simulink model "Lombardini_dual_fuel"  (R2024b)
settings: Solver=FixedStepAuto  StartTime=0.0  StopTime=2000  RelTol=1e-3  EnableMultiTasking=on
PreLoadFcn:
  | try, eval([bdroot '_setup']); catch, eval('model_setup', ''); end
InitFcn:
  | try, eval([bdroot '_setup']); catch, eval('model_setup', ''); end
model workspace (MAT data in the model file):
  PID_rpm = [1000 2000 3000 4000]
undefined symbols (not defined in the file): ECU555, motohawk_build_version, motohawk_get_target_image, motohawk_target_type, motohawk_trunc_name, motohawk_vardec_path
libraries: MotoHawk_lib x118, motohawk_annotations_lib x23, dspstat3 x13, motohawk_examples_lib x1, MotoHawk_Protocols_lib x1
(part 3 of 5)

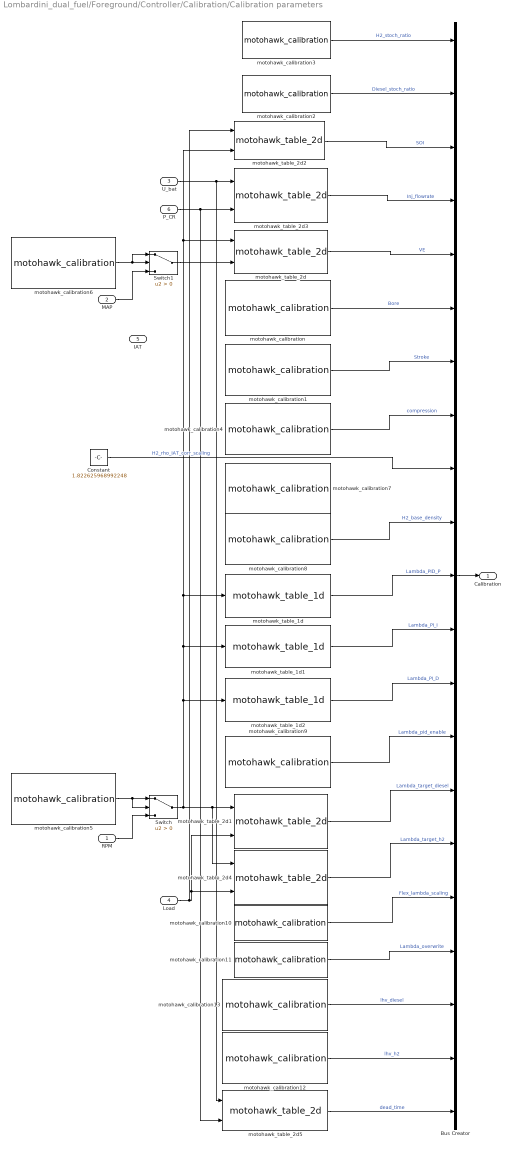
== system Lombardini_dual_fuel/Foreground/Controller/Calibration/Calibration parameters ==
  RPM : Inport
  MAP : Inport  Port=2
  U_bat : Inport  Port=3
  Load : Inport  Port=4
  IAT : Inport  Port=5
  P_CR : Inport  Port=6
  Bus Creator : BusCreator  Inputs=21
  Constant : Constant  Value=1.822625968992248
  Switch : Switch  Criteria=u2 > Threshold  SaturateOnIntegerOverflow=off  InputSameDT=off
  Switch1 : Switch  Criteria=u2 > Threshold  SaturateOnIntegerOverflow=off  InputSameDT=off
  motohawk_calibration : MotoHawk_lib/Calibration & Probing Blocks/motohawk_calibration  name_source=Use Parameter  nam='Bore'  val=69  storage=Calibration  ovr_cals=on  data_type=Inherit from 'Default Value'  mem_region_use=off  mem_region_name='SERIAL_EE'  read_level=1  write_level=1  view_as=Number  enum_struct={'Disabled', 'Enabled'}  vector_style=Wide Row  row_header_enum={}  col_header_enum={}  mototune_group=motohawk_vardec_path(gcb)  help=''  units=''  min_val=-inf  max_val=inf  precision=''  gain=1  offset=0  exp=1  show_more=on  use_help_units=on  use_header_enum=off  use_min_max=off  use_precision=off  use_mototune_group=on  data_stores=motohawk_sfun_calibration_data_stores
      settings: SourceProductName=MotoHawk
  motohawk_calibration1 : MotoHawk_lib/Calibration & Probing Blocks/motohawk_calibration  name_source=Use Parameter  nam='Stroke'  val=64  storage=Calibration  ovr_cals=on  data_type=Inherit from 'Default Value'  mem_region_use=off  mem_region_name='SERIAL_EE'  read_level=1  write_level=1  view_as=Number  enum_struct={'Disabled', 'Enabled'}  vector_style=Wide Row  row_header_enum={}  col_header_enum={}  mototune_group=motohawk_vardec_path(gcb)  help=''  units=''  min_val=-inf  max_val=inf  precision=''  gain=1  offset=0  exp=1  show_more=on  use_help_units=on  use_header_enum=off  use_min_max=off  use_precision=off  use_mototune_group=on  data_stores=motohawk_sfun_calibration_data_stores
      settings: SourceProductName=MotoHawk
  motohawk_calibration10 : MotoHawk_lib/Calibration & Probing Blocks/motohawk_calibration  name_source=Use Parameter  nam='Flex_lambda_scaling'  val=1  storage=Calibration  ovr_cals=on  data_type=Inherit from 'Default Value'  mem_region_use=off  mem_region_name='SERIAL_EE'  read_level=1  write_level=1  view_as=Number  enum_struct={'Disabled', 'Enabled'}  vector_style=Wide Row  row_header_enum={}  col_header_enum={}  mototune_group=motohawk_vardec_path(gcb)  help=''  units=''  min_val=-inf  max_val=inf  precision=''  gain=1  offset=0  exp=1  show_more=off  use_help_units=off  use_header_enum=off  use_min_max=off  use_precision=off  use_mototune_group=off  data_stores=motohawk_sfun_calibration_data_stores
      settings: SourceProductName=MotoHawk
  motohawk_calibration11 : MotoHawk_lib/Calibration & Probing Blocks/motohawk_calibration  name_source=Use Parameter  nam='Lambda_Overwrite'  val=0  storage=Calibration  ovr_cals=on  data_type=Inherit from 'Default Value'  mem_region_use=off  mem_region_name='SERIAL_EE'  read_level=1  write_level=1  view_as=Number  enum_struct={'Disabled', 'Enabled'}  vector_style=Wide Row  row_header_enum={}  col_header_enum={}  mototune_group=motohawk_vardec_path(gcb)  help=''  units=''  min_val=-inf  max_val=inf  precision=''  gain=1  offset=0  exp=1  show_more=off  use_help_units=off  use_header_enum=off  use_min_max=off  use_precision=off  use_mototune_group=off  data_stores=motohawk_sfun_calibration_data_stores
      settings: SourceProductName=MotoHawk
  motohawk_calibration12 : MotoHawk_lib/Calibration & Probing Blocks/motohawk_calibration  name_source=Use Parameter  nam='LHV_H2'  val=120000  storage=Calibration  ovr_cals=on  data_type=Inherit from 'Default Value'  mem_region_use=off  mem_region_name='SERIAL_EE'  read_level=1  write_level=1  view_as=Number  enum_struct={'Disabled', 'Enabled'}  vector_style=Wide Row  row_header_enum={}  col_header_enum={}  mototune_group=motohawk_vardec_path(gcb)  help=''  units=''  min_val=-inf  max_val=inf  precision=''  gain=1  offset=0  exp=1  show_more=on  use_help_units=on  use_header_enum=off  use_min_max=off  use_precision=off  use_mototune_group=on  data_stores=motohawk_sfun_calibration_data_stores
      settings: SourceProductName=MotoHawk
  motohawk_calibration13 : MotoHawk_lib/Calibration & Probing Blocks/motohawk_calibration  name_source=Use Parameter  nam='LHV_Diesel'  val=42800  storage=Calibration  ovr_cals=on  data_type=Inherit from 'Default Value'  mem_region_use=off  mem_region_name='SERIAL_EE'  read_level=1  write_level=1  view_as=Number  enum_struct={'Disabled', 'Enabled'}  vector_style=Wide Row  row_header_enum={}  col_header_enum={}  mototune_group=motohawk_vardec_path(gcb)  help=''  units=''  min_val=-inf  max_val=inf  precision=''  gain=1  offset=0  exp=1  show_more=on  use_help_units=on  use_header_enum=off  use_min_max=off  use_precision=off  use_mototune_group=on  data_stores=motohawk_sfun_calibration_data_stores
      settings: SourceProductName=MotoHawk
  motohawk_calibration2 : MotoHawk_lib/Calibration & Probing Blocks/motohawk_calibration  name_source=Use Parameter  nam='Diesel_Stoch_ratio'  val=14.7  storage=Calibration  ovr_cals=on  data_type=Inherit from 'Default Value'  mem_region_use=off  mem_region_name='SERIAL_EE'  read_level=1  write_level=1  view_as=Number  enum_struct={'Disabled', 'Enabled'}  vector_style=Wide Row  row_header_enum={}  col_header_enum={}  mototune_group=motohawk_vardec_path(gcb)  help=''  units=''  min_val=-inf  max_val=inf  precision=''  gain=1  offset=0  exp=1  show_more=off  use_help_units=off  use_header_enum=off  use_min_max=off  use_precision=off  use_mototune_group=off  data_stores=motohawk_sfun_calibration_data_stores
      settings: SourceProductName=MotoHawk
  motohawk_calibration3 : MotoHawk_lib/Calibration & Probing Blocks/motohawk_calibration  name_source=Use Parameter  nam='H2_Stoch_ratio'  val=34.3  storage=Calibration  ovr_cals=on  data_type=Inherit from 'Default Value'  mem_region_use=off  mem_region_name='SERIAL_EE'  read_level=1  write_level=1  view_as=Number  enum_struct={'Disabled', 'Enabled'}  vector_style=Wide Row  row_header_enum={}  col_header_enum={}  mototune_group=motohawk_vardec_path(gcb)  help=''  units=''  min_val=-inf  max_val=inf  precision=''  gain=1  offset=0  exp=1  show_more=off  use_help_units=off  use_header_enum=off  use_min_max=off  use_precision=off  use_mototune_group=off  data_stores=motohawk_sfun_calibration_data_stores
      settings: SourceProductName=MotoHawk
  motohawk_calibration4 : MotoHawk_lib/Calibration & Probing Blocks/motohawk_calibration  name_source=Use Parameter  nam='Compression'  val=20  storage=Calibration  ovr_cals=on  data_type=Inherit from 'Default Value'  mem_region_use=off  mem_region_name='SERIAL_EE'  read_level=1  write_level=1  view_as=Number  enum_struct={'Disabled', 'Enabled'}  vector_style=Wide Row  row_header_enum={}  col_header_enum={}  mototune_group=motohawk_vardec_path(gcb)  help=''  units=''  min_val=-inf  max_val=inf  precision=''  gain=1  offset=0  exp=1  show_more=on  use_help_units=on  use_header_enum=off  use_min_max=off  use_precision=off  use_mototune_group=on  data_stores=motohawk_sfun_calibration_data_stores
      settings: SourceProductName=MotoHawk
  motohawk_calibration5 : MotoHawk_lib/Calibration & Probing Blocks/motohawk_calibration  name_source=Use Parameter  nam='RPM_Overwrite'  val=0  storage=Calibration  ovr_cals=on  data_type=Inherit from 'Default Value'  mem_region_use=off  mem_region_name='SERIAL_EE'  read_level=1  write_level=1  view_as=Number  enum_struct={'Disabled', 'Enabled'}  vector_style=Wide Row  row_header_enum={}  col_header_enum={}  mototune_group=motohawk_vardec_path(gcb)  help=''  units=''  min_val=-inf  max_val=inf  precision=''  gain=1  offset=0  exp=1  show_more=on  use_help_units=on  use_header_enum=off  use_min_max=off  use_precision=off  use_mototune_group=on  data_stores=motohawk_sfun_calibration_data_stores
      settings: SourceProductName=MotoHawk
  motohawk_calibration6 : MotoHawk_lib/Calibration & Probing Blocks/motohawk_calibration  name_source=Use Parameter  nam='MAP_Overwrite'  val=0  storage=Calibration  ovr_cals=on  data_type=Inherit from 'Default Value'  mem_region_use=off  mem_region_name='SERIAL_EE'  read_level=1  write_level=1  view_as=Number  enum_struct={'Disabled', 'Enabled'}  vector_style=Wide Row  row_header_enum={}  col_header_enum={}  mototune_group=motohawk_vardec_path(gcb)  help=''  units=''  min_val=-inf  max_val=inf  precision=''  gain=1  offset=0  exp=1  show_more=on  use_help_units=on  use_header_enum=off  use_min_max=off  use_precision=off  use_mototune_group=on  data_stores=motohawk_sfun_calibration_data_stores
      settings: SourceProductName=MotoHawk
  motohawk_calibration7 : MotoHawk_lib/Calibration & Probing Blocks/motohawk_calibration  name_source=Use Parameter  nam='H2_rho_IAT_corr_gain'  val=1.5  storage=Calibration  ovr_cals=on  data_type=Inherit from 'Default Value'  mem_region_use=off  mem_region_name='SERIAL_EE'  read_level=1  write_level=1  view_as=Number  enum_struct={'Disabled', 'Enabled'}  vector_style=Wide Row  row_header_enum={}  col_header_enum={}  mototune_group=motohawk_vardec_path(gcb)  help=''  units=''  min_val=-inf  max_val=inf  precision=''  gain=1  offset=0  exp=1  show_more=on  use_help_units=on  use_header_enum=off  use_min_max=off  use_precision=off  use_mototune_group=on  data_stores=motohawk_sfun_calibration_data_stores
      settings: SourceProductName=MotoHawk
  motohawk_calibration8 : MotoHawk_lib/Calibration & Probing Blocks/motohawk_calibration  name_source=Use Parameter  nam='H2_base_density'  val=0.00008988  storage=Calibration  ovr_cals=on  data_type=Inherit from 'Default Value'  mem_region_use=off  mem_region_name='SERIAL_EE'  read_level=1  write_level=1  view_as=Number  enum_struct={'Disabled', 'Enabled'}  vector_style=Wide Row  row_header_enum={}  col_header_enum={}  mototune_group=motohawk_vardec_path(gcb)  help=''  units=''  min_val=-inf  max_val=inf  precision=''  gain=1  offset=0  exp=1  show_more=on  use_help_units=on  use_header_enum=off  use_min_max=off  use_precision=off  use_mototune_group=on  data_stores=motohawk_sfun_calibration_data_stores
      settings: SourceProductName=MotoHawk
  motohawk_calibration9 : MotoHawk_lib/Calibration & Probing Blocks/motohawk_calibration  name_source=Use Parameter  nam='Lambda_pid_enable'  val=0  storage=Calibration  ovr_cals=on  data_type=Inherit from 'Default Value'  mem_region_use=off  mem_region_name='SERIAL_EE'  read_level=1  write_level=1  view_as=Number  enum_struct={'Disabled', 'Enabled'}  vector_style=Wide Row  row_header_enum={}  col_header_enum={}  mototune_group=motohawk_vardec_path(gcb)  help=''  units=''  min_val=-inf  max_val=inf  precision=''  gain=1  offset=0  exp=1  show_more=on  use_help_units=on  use_header_enum=off  use_min_max=off  use_precision=off  use_mototune_group=on  data_stores=motohawk_sfun_calibration_data_stores
      settings: SourceProductName=MotoHawk
  motohawk_table_1d : MotoHawk_lib/Lookup Tables/motohawk_table_1d  nam='Lambda_PID_P'  bp_nam=''  breakpoint_data=PID_rpm  bp_data_type=Inherit from 'Breakpoint Data'  table_data=[0.5 0.5 0.5 0.5]  table_data_type=Inherit from 'Table Data'  out_type=Inherit from 'Table Data'  input_name=''  output_name=''  bp_storage=Constant  bp_mem_region_use=off  bp_mem_region_name='SERIAL_EE'  storage=NonAdaptive  mem_region_use=off  mem_region_name='SERIAL_EE'  read_level=1  write_level=1  ovr_cals=on  mototune_group=motohawk_vardec_path(gcb)  help=''  bp_units=''  table_units=''  bp_min_val=-inf  bp_max_val=inf  min_val=-inf  max_val=inf  b_precision=''  b_gain=1  b_offset=0  b_exp=1  t_precision=''  t_gain=1  t_offset=0  t_exp=1  show_more=on  use_help=off  use_min_max=off  use_precision=off  use_breakpoint=off  use_table=off  use_links=off  use_mototune_group=off  data_stores=motohawk_table_1d_data_stores
      settings: SourceProductName=MotoHawk
  motohawk_table_1d1 : MotoHawk_lib/Lookup Tables/motohawk_table_1d  nam='Lambda_PID_I'  bp_nam=''  breakpoint_data=PID_rpm  bp_data_type=Inherit from 'Breakpoint Data'  table_data=[0.5 0.5 0.5 0.5 ]  table_data_type=Inherit from 'Table Data'  out_type=Inherit from 'Table Data'  input_name=''  output_name=''  bp_storage=Constant  bp_mem_region_use=off  bp_mem_region_name='SERIAL_EE'  storage=NonAdaptive  mem_region_use=off  mem_region_name='SERIAL_EE'  read_level=1  write_level=1  ovr_cals=on  mototune_group=motohawk_vardec_path(gcb)  help=''  bp_units=''  table_units=''  bp_min_val=-inf  bp_max_val=inf  min_val=-inf  max_val=inf  b_precision=''  b_gain=1  b_offset=0  b_exp=1  t_precision=''  t_gain=1  t_offset=0  t_exp=1  show_more=on  use_help=off  use_min_max=off  use_precision=off  use_breakpoint=off  use_table=off  use_links=off  use_mototune_group=off  data_stores=motohawk_table_1d_data_stores
      settings: SourceProductName=MotoHawk
  motohawk_table_1d2 : MotoHawk_lib/Lookup Tables/motohawk_table_1d  nam='Lambda_PID_D'  bp_nam=''  breakpoint_data=PID_rpm  bp_data_type=Inherit from 'Breakpoint Data'  table_data=[ 0 0 0 0]  table_data_type=Inherit from 'Table Data'  out_type=Inherit from 'Table Data'  input_name=''  output_name=''  bp_storage=Constant  bp_mem_region_use=off  bp_mem_region_name='SERIAL_EE'  storage=NonAdaptive  mem_region_use=off  mem_region_name='SERIAL_EE'  read_level=1  write_level=1  ovr_cals=on  mototune_group=motohawk_vardec_path(gcb)  help=''  bp_units=''  table_units=''  bp_min_val=-inf  bp_max_val=inf  min_val=-inf  max_val=inf  b_precision=''  b_gain=1  b_offset=0  b_exp=1  t_precision=''  t_gain=1  t_offset=0  t_exp=1  show_more=on  use_help=off  use_min_max=off  use_precision=off  use_breakpoint=off  use_table=off  use_links=off  use_mototune_group=off  data_stores=motohawk_table_1d_data_stores
      settings: SourceProductName=MotoHawk
  motohawk_table_2d : MotoHawk_lib/Lookup Tables/motohawk_table_2d  nam='VE_Table'  row_breakpoint_data=1500:500:4000  col_breakpoint_data=[0 1.5 2.5 3]  table_data=[64 64 64 64; 67 67 67 67; 80 80 80 80; 77 77 77 77; 79 79 79 79; 81 81 81 81]  row_bp_data_type=Inherit from 'Row Breakpoint Data'  col_bp_data_type=Inherit from 'Column Breakpoint Data'  table_data_type=Inherit from 'Table Data'  out_type=Inherit from 'Table Data'  row_nam=''  col_nam=''  row_input_name=''  col_input_name=''  output_name=''  bp_storage=Constant  bp_mem_region_use=off  bp_mem_region_name='SERIAL_EE'  storage=NonAdaptive  mem_region_use=off  mem_region_name='SERIAL_EE'  read_level=1  write_level=1  ovr_cals=on  mototune_group=motohawk_vardec_path(gcb)  help=''  row_bp_units=''  col_bp_units=''  table_units=''  row_bp_min_val=-inf  row_bp_max_val=inf  col_bp_min_val=-inf  col_bp_max_val=inf  min_val=-inf  max_val=inf  rb_precision=''  rb_gain=1  rb_offset=0  rb_exp=1  cb_precision=''  cb_gain=1  cb_offset=0  cb_exp=1  t_precision=''  t_gain=1  t_offset=0  t_exp=1  show_more=off  use_help=off  use_min_max=off  use_precision=off  use_row_breakpoint=off  use_col_breakpoint=off  use_table=off  use_links=off  use_mototune_group=off  data_stores=motohawk_table_2d_data_stores
      settings: SourceProductName=MotoHawk
  motohawk_table_2d1 : MotoHawk_lib/Lookup Tables/motohawk_table_2d  nam='Lambda_target_diesel'  row_breakpoint_data=1500:500:5000  col_breakpoint_data=0:10:100  table_data=repmat(linspace(5, 1.3, 11), 8, 1)  row_bp_data_type=Inherit from 'Row Breakpoint Data'  col_bp_data_type=Inherit from 'Column Breakpoint Data'  table_data_type=Inherit from 'Table Data'  out_type=Inherit from 'Table Data'  row_nam=''  col_nam=''  row_input_name=''  col_input_name=''  output_name=''  bp_storage=Constant  bp_mem_region_use=off  bp_mem_region_name='SERIAL_EE'  storage=NonAdaptive  mem_region_use=off  mem_region_name='SERIAL_EE'  read_level=1  write_level=1  ovr_cals=on  mototune_group=motohawk_vardec_path(gcb)  help=''  row_bp_units=''  col_bp_units=''  table_units=''  row_bp_min_val=-inf  row_bp_max_val=inf  col_bp_min_val=-inf  col_bp_max_val=inf  min_val=-inf  max_val=inf  rb_precision=''  rb_gain=1  rb_offset=0  rb_exp=1  cb_precision=''  cb_gain=1  cb_offset=0  cb_exp=1  t_precision=''  t_gain=1  t_offset=0  t_exp=1  show_more=off  use_help=off  use_min_max=off  use_precision=off  use_row_breakpoint=off  use_col_breakpoint=off  use_table=off  use_links=off  use_mototune_group=off  data_stores=motohawk_table_2d_data_stores
      settings: SourceProductName=MotoHawk
  motohawk_table_2d2 : MotoHawk_lib/Lookup Tables/motohawk_table_2d  nam='SOI'  row_breakpoint_data=[0 1 2 3 4 5 6 7 8 9]  col_breakpoint_data=[0 1 2 3 4 5 6 7 8 9]  table_data=zeros(10)  row_bp_data_type=Inherit from 'Row Breakpoint Data'  col_bp_data_type=Inherit from 'Column Breakpoint Data'  table_data_type=Inherit from 'Table Data'  out_type=Inherit from 'Table Data'  row_nam=''  col_nam=''  row_input_name=''  col_input_name=''  output_name=''  bp_storage=Constant  bp_mem_region_use=off  bp_mem_region_name='SERIAL_EE'  storage=NonAdaptive  mem_region_use=off  mem_region_name='SERIAL_EE'  read_level=1  write_level=1  ovr_cals=on  mototune_group=motohawk_vardec_path(gcb)  help=''  row_bp_units=''  col_bp_units=''  table_units=''  row_bp_min_val=-inf  row_bp_max_val=inf  col_bp_min_val=-inf  col_bp_max_val=inf  min_val=-inf  max_val=inf  rb_precision=''  rb_gain=1  rb_offset=0  rb_exp=1  cb_precision=''  cb_gain=1  cb_offset=0  cb_exp=1  t_precision=''  t_gain=1  t_offset=0  t_exp=1  show_more=off  use_help=off  use_min_max=off  use_precision=off  use_row_breakpoint=off  use_col_breakpoint=off  use_table=off  use_links=off  use_mototune_group=off  data_stores=motohawk_table_2d_data_stores
      settings: SourceProductName=MotoHawk
  motohawk_table_2d3 : MotoHawk_lib/Lookup Tables/motohawk_table_2d  nam='Inj_flowrate_P_CR_corr'  row_breakpoint_data=[200 400 600 800 1000 1200 1400 1600 1800]  col_breakpoint_data=[11 13.5 15]  table_data=|  row_bp_data_type=Inherit from 'Row Breakpoint Data'  col_bp_data_type=Inherit from 'Column Breakpoint Data'  table_data_type=Inherit from 'Table Data'  out_type=Inherit from 'Table Data'  row_nam=''  col_nam=''  row_input_name=''  col_input_name=''  output_name=''  bp_storage=Constant  bp_mem_region_use=off  bp_mem_region_name='SERIAL_EE'  storage=NonAdaptive  mem_region_use=off  mem_region_name='SERIAL_EE'  read_level=1  write_level=1  ovr_cals=on  mototune_group=motohawk_vardec_path(gcb)  help=''  row_bp_units=''  col_bp_units=''  table_units=''  row_bp_min_val=-inf  row_bp_max_val=inf  col_bp_min_val=-inf  col_bp_max_val=inf  min_val=-inf  max_val=inf  rb_precision=''  rb_gain=1  rb_offset=0  rb_exp=1  cb_precision=''  cb_gain=1  cb_offset=0  cb_exp=1  t_precision=''  t_gain=1  t_offset=0  t_exp=1  show_more=off  use_help=off  use_min_max=off  use_precision=off  use_row_breakpoint=off  use_col_breakpoint=off  use_table=off  use_links=off  use_mototune_group=off  data_stores=motohawk_table_2d_data_stores
      | [ 25   28   30;
      |     42   46   49;
      |     58   63   66;
      |     72   78   82;
      |     85   92   97;
      |     95  103  108;
      |     104 112  118;
      |     112 121  127;
      |     119 129  135
      | ]
      settings: SourceProductName=MotoHawk
  motohawk_table_2d4 : MotoHawk_lib/Lookup Tables/motohawk_table_2d  nam='Lambda_target_H2'  row_breakpoint_data=1500:500:5000  col_breakpoint_data=0:10:100  table_data=repmat(linspace(5, 1.3, 11), 8, 1)  row_bp_data_type=Inherit from 'Row Breakpoint Data'  col_bp_data_type=Inherit from 'Column Breakpoint Data'  table_data_type=Inherit from 'Table Data'  out_type=Inherit from 'Table Data'  row_nam=''  col_nam=''  row_input_name=''  col_input_name=''  output_name=''  bp_storage=Constant  bp_mem_region_use=off  bp_mem_region_name='SERIAL_EE'  storage=NonAdaptive  mem_region_use=off  mem_region_name='SERIAL_EE'  read_level=1  write_level=1  ovr_cals=on  mototune_group=motohawk_vardec_path(gcb)  help=''  row_bp_units=''  col_bp_units=''  table_units=''  row_bp_min_val=-inf  row_bp_max_val=inf  col_bp_min_val=-inf  col_bp_max_val=inf  min_val=-inf  max_val=inf  rb_precision=''  rb_gain=1  rb_offset=0  rb_exp=1  cb_precision=''  cb_gain=1  cb_offset=0  cb_exp=1  t_precision=''  t_gain=1  t_offset=0  t_exp=1  show_more=off  use_help=off  use_min_max=off  use_precision=off  use_row_breakpoint=off  use_col_breakpoint=off  use_table=off  use_links=off  use_mototune_group=off  data_stores=motohawk_table_2d_data_stores
      settings: SourceProductName=MotoHawk
  motohawk_table_2d5 : MotoHawk_lib/Lookup Tables/motohawk_table_2d  nam='Dead_time_table'  row_breakpoint_data=[0 1 2 3 4 5 6 7 8 9 ]  col_breakpoint_data=[0 1 2 3 4 5 6 7 8 9 ]  table_data=zeros(10)  row_bp_data_type=Inherit from 'Row Breakpoint Data'  col_bp_data_type=Inherit from 'Column Breakpoint Data'  table_data_type=Inherit from 'Table Data'  out_type=Inherit from 'Table Data'  row_nam=''  col_nam=''  row_input_name=''  col_input_name=''  output_name=''  bp_storage=Constant  bp_mem_region_use=off  bp_mem_region_name='SERIAL_EE'  storage=NonAdaptive  mem_region_use=off  mem_region_name='SERIAL_EE'  read_level=1  write_level=1  ovr_cals=on  mototune_group=motohawk_vardec_path(gcb)  help=''  row_bp_units=''  col_bp_units=''  table_units=''  row_bp_min_val=-inf  row_bp_max_val=inf  col_bp_min_val=-inf  col_bp_max_val=inf  min_val=-inf  max_val=inf  rb_precision=''  rb_gain=1  rb_offset=0  rb_exp=1  cb_precision=''  cb_gain=1  cb_offset=0  cb_exp=1  t_precision=''  t_gain=1  t_offset=0  t_exp=1  show_more=off  use_help=off  use_min_max=off  use_precision=off  use_row_breakpoint=off  use_col_breakpoint=off  use_table=off  use_links=off  use_mototune_group=off  data_stores=motohawk_table_2d_data_stores
      settings: SourceProductName=MotoHawk
  Calibration : Outport
  wires:
  motohawk_calibration/1 -> Bus Creator/6  "Bore"
  U_bat/1 -> motohawk_table_2d5/1, motohawk_table_2d3/1
  motohawk_table_1d1/1 -> Bus Creator/12  "Lambda_PI_I"
  motohawk_calibration4/1 -> Bus Creator/8  "compression"
  MAP/1 -> Switch1/3
  motohawk_calibration6/1 -> Switch1/1, Switch1/2
  Switch1/1 -> motohawk_table_2d/2
  motohawk_calibration1/1 -> Bus Creator/7  "Stroke"
  P_CR/1 -> motohawk_table_2d5/2, motohawk_table_2d3/2
  motohawk_table_1d/1 -> Bus Creator/11  "Lambda_PID_P"
  motohawk_calibration3/1 -> Bus Creator/1  "H2_stoch_ratio"
  RPM/1 -> Switch/3
  motohawk_calibration5/1 -> Switch/2, Switch/1
  motohawk_calibration11/1 -> Bus Creator/18  "Lambda_overwrite"
  Switch/1 -> motohawk_table_2d1/1, motohawk_table_2d4/1, motohawk_table_2d2/2, motohawk_table_2d/1, motohawk_table_1d/1, motohawk_table_1d1/1, motohawk_table_1d2/1
  motohawk_calibration2/1 -> Bus Creator/2  "Diesel_stoch_ratio"
  Load/1 -> motohawk_table_2d1/2, motohawk_table_2d4/2, motohawk_table_2d2/1
  motohawk_calibration10/1 -> Bus Creator/17  "Flex_lambda_scaling"
  motohawk_table_2d2/1 -> Bus Creator/3  "SOI"
  motohawk_table_2d3/1 -> Bus Creator/4  "Inj_flowrate"
  motohawk_table_2d/1 -> Bus Creator/5  "VE"
  motohawk_calibration8/1 -> Bus Creator/10  "H2_base_density"
  motohawk_table_1d2/1 -> Bus Creator/13  "Lambda_PI_D"
  Bus Creator/1 -> Calibration/1
  motohawk_calibration9/1 -> Bus Creator/14  "Lambda_pid_enable"
  motohawk_table_2d1/1 -> Bus Creator/15  "Lambda_target_diesel"
  motohawk_table_2d4/1 -> Bus Creator/16  "Lambda_target_h2"
  motohawk_calibration13/1 -> Bus Creator/19  "lhv_diesel"
  motohawk_calibration12/1 -> Bus Creator/20  "lhv_h2"
  motohawk_table_2d5/1 -> Bus Creator/21  "dead_time"
  Constant/1 -> Bus Creator/9  "H2_rho_IAT_corr_scaling"

== system Lombardini_dual_fuel/Foreground/Controller/Controller/CR Pressure control ==
  Load : Inport
  RPM : Inport  Port=2
  <P_CR> : Inport  Port=3
  Add : Sum
  Add1 : Sum
  I : Gain
  P : Gain
  Subtract : Sum  Inputs=+-
  motohawk_table_2d : MotoHawk_lib/Lookup Tables/motohawk_table_2d  nam='CR_p_target'  row_breakpoint_data=[0 1.5 2]  col_breakpoint_data=[0 1.5 2.5 3]  table_data=[11 12 13 14; 21 22 23 24; 31 32 33 34]  row_bp_data_type=Inherit from 'Row Breakpoint Data'  col_bp_data_type=Inherit from 'Column Breakpoint Data'  table_data_type=Inherit from 'Table Data'  out_type=Inherit from 'Table Data'  row_nam=''  col_nam=''  row_input_name=''  col_input_name=''  output_name=''  bp_storage=Constant  bp_mem_region_use=off  bp_mem_region_name='SERIAL_EE'  storage=NonAdaptive  mem_region_use=off  mem_region_name='SERIAL_EE'  read_level=1  write_level=1  ovr_cals=on  mototune_group=motohawk_vardec_path(gcb)  help=''  row_bp_units=''  col_bp_units=''  table_units=''  row_bp_min_val=-inf  row_bp_max_val=inf  col_bp_min_val=-inf  col_bp_max_val=inf  min_val=-inf  max_val=inf  rb_precision=''  rb_gain=1  rb_offset=0  rb_exp=1  cb_precision=''  cb_gain=1  cb_offset=0  cb_exp=1  t_precision=''  t_gain=1  t_offset=0  t_exp=1  show_more=off  use_help=off  use_min_max=off  use_precision=off  use_row_breakpoint=off  use_col_breakpoint=off  use_table=off  use_links=off  use_mototune_group=off  data_stores=motohawk_table_2d_data_stores
      settings: SourceProductName=MotoHawk
  P_CR_Res : Outport
  wires:
  Load/1 -> motohawk_table_2d/1
  RPM/1 -> motohawk_table_2d/2
  <P_CR>/1 -> Subtract/1
  motohawk_table_2d/1 -> Subtract/2, Add/2
  Add/1 -> P_CR_Res/1
  P/1 -> Add1/1
  I/1 -> Add1/2
  Subtract/1 -> P/1, I/1
  Add1/1 -> Add/1
